simulink model "Schema_fonctionnel"  (R2020b)
settings: Solver=VariableStepAuto  StartTime=0.0  StopTime=10.0  RelTol=1e-3
settings Model: Creator=vince  LastModifiedBy=Roxanne Simard

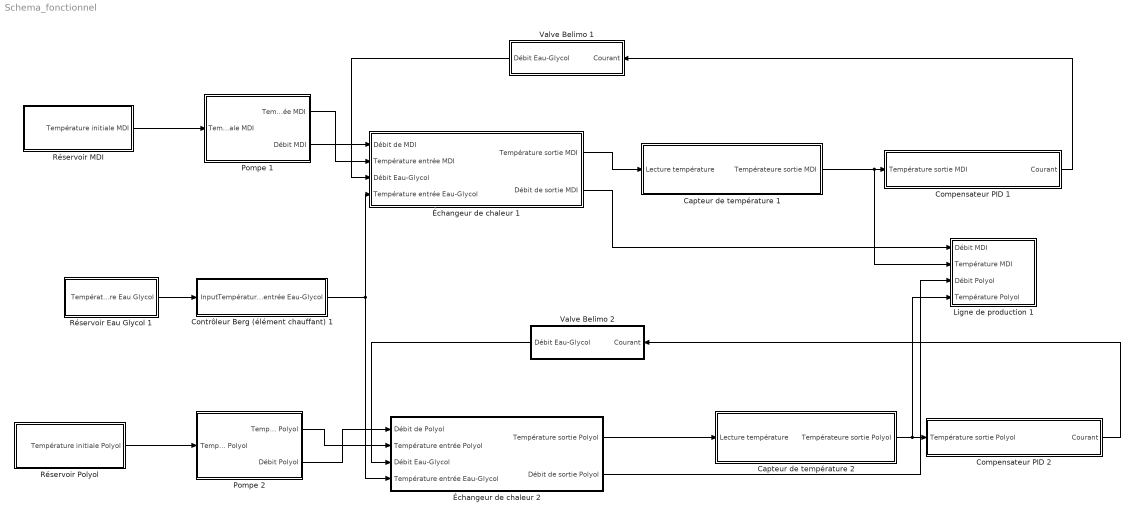
== system Schema_fonctionnel ==
  Capteur de température 1 : Subsystem
  Capteur de température 2 : Subsystem
  Compensateur PID 1 : Subsystem
  Compensateur PID 2 : Subsystem
  Contrôleur Berg (élément chauffant) 1 : Subsystem
  Ligne de production 1 : Subsystem
  Pompe 1 : Subsystem
  Pompe 2 : Subsystem
  Réservoir Eau Glycol 1 : Subsystem
  Réservoir MDI : Subsystem
  Réservoir Polyol : Subsystem
  Valve Belimo 1 : Subsystem
  Valve Belimo 2 : Subsystem
  Échangeur de chaleur 1 : Subsystem
  Échangeur de chaleur 2 : Subsystem
  wires:
  Échangeur de chaleur 1/1(Température sortie MDI) -> Capteur de température 1/1(Lecture température)
  Capteur de température 1/1(Températeure sortie MDI) -> Ligne de production 1/2(Température MDI), Compensateur PID 1/1(Température sortie MDI)
  Échangeur de chaleur 1/2(Débit de sortie MDI) -> Ligne de production 1/1(Débit MDI)
  Compensateur PID 1/1(Courant) -> Valve Belimo 1/1(Courant)
  Valve Belimo 1/1(Débit Eau-Glycol) -> Échangeur de chaleur 1/3(Débit Eau-Glycol)
  Réservoir MDI/1(Température initiale MDI) -> Pompe 1/1(Température initiale MDI)
  Pompe 1/2(Débit MDI) -> Échangeur de chaleur 1/1(Débit de MDI)
  Pompe 1/1(Température entrée MDI) -> Échangeur de chaleur 1/2(Température entrée MDI)
  Réservoir Eau Glycol 1/1(Température Eau Glycol) -> Contrôleur Berg (élément chauffant) 1/1(Input)
  Contrôleur Berg (élément chauffant) 1/1(Température entrée Eau-Glycol) -> Échangeur de chaleur 2/4(Température entrée Eau-Glycol), Échangeur de chaleur 1/4(Température entrée Eau-Glycol)
  Valve Belimo 2/1(Débit Eau-Glycol) -> Échangeur de chaleur 2/3(Débit Eau-Glycol)
  Réservoir Polyol/1(Température initiale Polyol) -> Pompe 2/1(Température initiale Polyol)
  Capteur de température 2/1(Températeure sortie Polyol) -> Ligne de production 1/4(Température Polyol), Compensateur PID 2/1(Température sortie Polyol)
  Pompe 2/2(Débit Polyol) -> Échangeur de chaleur 2/1(Débit de Polyol)
  Échangeur de chaleur 2/2(Débit de sortie Polyol) -> Ligne de production 1/3(Débit Polyol)
  Pompe 2/1(Température entrée Polyol) -> Échangeur de chaleur 2/2(Température entrée Polyol)
  Échangeur de chaleur 2/1(Température sortie Polyol) -> Capteur de température 2/1(Lecture température)
  Compensateur PID 2/1(Courant) -> Valve Belimo 2/1(Courant)

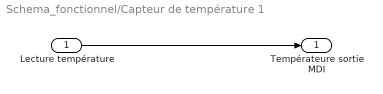
== system Schema_fonctionnel/Capteur de température 1 ==
  Lecture température : Inport
  Températeure sortie MDI : Outport
  wires:
  Lecture température/1 -> Températeure sortie MDI/1

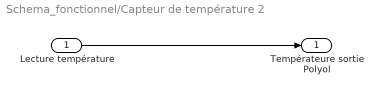
== system Schema_fonctionnel/Capteur de température 2 ==
  Lecture température : Inport
  Températeure sortie Polyol : Outport
  wires:
  Lecture température/1 -> Températeure sortie Polyol/1

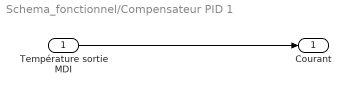
== system Schema_fonctionnel/Compensateur PID 1 ==
  Température sortie MDI : Inport
  Courant : Outport
  wires:
  Température sortie MDI/1 -> Courant/1

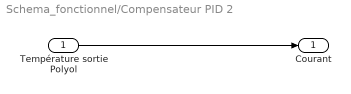
== system Schema_fonctionnel/Compensateur PID 2 ==
  Température sortie Polyol : Inport
  Courant : Outport
  wires:
  Température sortie Polyol/1 -> Courant/1

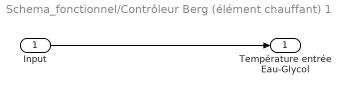
== system Schema_fonctionnel/Contrôleur Berg (élément chauffant) 1 ==
  Input : Inport
  Température entrée Eau-Glycol : Outport
  wires:
  Input/1 -> Température entrée Eau-Glycol/1

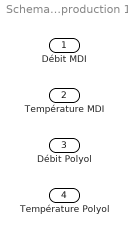
== system Schema_fonctionnel/Ligne de production 1 ==
  Débit MDI : Inport
  Température MDI : Inport  Port=2
  Débit Polyol : Inport  Port=3
  Température Polyol : Inport  Port=4

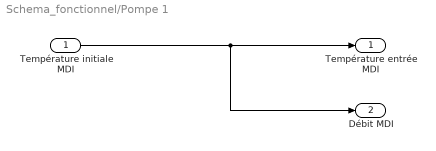
== system Schema_fonctionnel/Pompe 1 ==
  Température initiale MDI : Inport
  Température entrée MDI : Outport
  Débit MDI : Outport  Port=2
  wires:
  Température initiale MDI/1 -> Débit MDI/1, Température entrée MDI/1

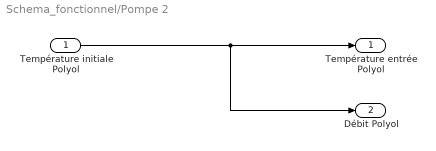
== system Schema_fonctionnel/Pompe 2 ==
  Température initiale Polyol : Inport
  Température entrée Polyol : Outport
  Débit Polyol : Outport  Port=2
  wires:
  Température initiale Polyol/1 -> Débit Polyol/1, Température entrée Polyol/1

== system Schema_fonctionnel/Réservoir Eau Glycol 1 ==
  Température Eau Glycol : Outport

== system Schema_fonctionnel/Réservoir MDI ==
  Température initiale MDI : Outport

== system Schema_fonctionnel/Réservoir Polyol ==
  Température initiale Polyol : Outport

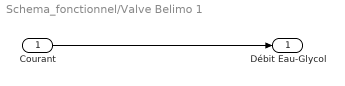
== system Schema_fonctionnel/Valve Belimo 1 ==
  Courant : Inport
  Débit Eau-Glycol : Outport
  wires:
  Courant/1 -> Débit Eau-Glycol/1

== system Schema_fonctionnel/Valve Belimo 2 ==
  Courant : Inport
  Débit Eau-Glycol : Outport
  wires:
  Courant/1 -> Débit Eau-Glycol/1

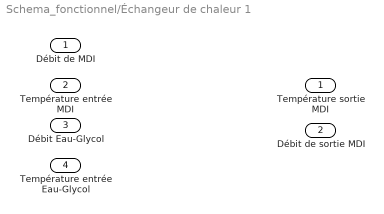
== system Schema_fonctionnel/Échangeur de chaleur 1 ==
  Débit de MDI : Inport
  Température entrée MDI : Inport  Port=2
  Débit Eau-Glycol : Inport  Port=3
  Température entrée Eau-Glycol : Inport  Port=4
  Température sortie MDI : Outport
  Débit de sortie MDI : Outport  Port=2

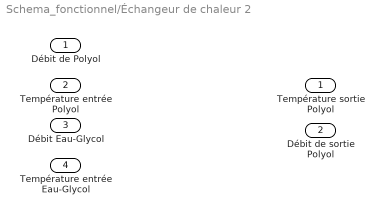
== system Schema_fonctionnel/Échangeur de chaleur 2 ==
  Débit de Polyol : Inport
  Température entrée Polyol : Inport  Port=2
  Débit Eau-Glycol : Inport  Port=3
  Température entrée Eau-Glycol : Inport  Port=4
  Température sortie Polyol : Outport
  Débit de sortie Polyol : Outport  Port=2
